simulink model "TAXI"  (R2024b)
settings: Solver=FixedStepDiscrete  StartTime=0.0  StopTime=13  FixedStep=0.01  RelTol=1e-3
settings Model: Creator=A  LastModifiedBy=A
settings OptimizationCC: DefaultParameterBehavior=Inlined  UseDivisionForNetSlopeComputation=on  GainParamInheritBuiltInType=on  UseFloatMulNetSlope=on  InlineInvariantSignals=on  ReuseModelBlockBuffer=off  PassReuseOutputArgsAs=Individual arguments  ZeroExternalMemoryAtStartup=off  ZeroInternalMemoryAtStartup=off  NoFixptDivByZeroProtection=on  EfficientFloat2IntCast=on  LifeSpan=1  OptimizeDataStoreBuffers=off  BusAssignmentInplaceUpdate=off  OptimizationLevel=level0  EfficientTunableParamExpr=on
settings DebuggingCC: ParameterTunabilityLossMsg=error  StrictBusMsg=ErrorOnBusTreatedAsVector  NonBusSignalsTreatedAsBus=error
settings HardwareCC: ProdBitPerPointer=32  ProdBitPerSizeT=32  ProdBitPerPtrDiffT=32  ProdLargestAtomicFloat=None  ProdWordSize=32  ProdLongLongMode=on  ProdHWDeviceType=Infineon->TriCore
settings SFSimCC: MATLABDynamicMemAlloc=off
settings RTWCC: Description=Embedded Coder  SystemTargetFile=ert.tlc  GenCodeOnly=on  TemplateMakefile=ert_default_tmf  GenerateReport=on  LaunchReport=on  DataTypeReplacement=CDataTypesFixedWidth  GenerateCodeMetricsReport=on
settings CodeAppCC: ForceParamTrailComments=on  IgnoreCustomStorageClasses=off  OperatorAnnotations=on  SimulinkDataObjDesc=on  SFDataObjDesc=on  CustomSymbolStrGlobalVar=rt$N$M  CustomSymbolStrType=$N$M  CustomSymbolStrFcn=$N$M$F  CustomSymbolStrMacro=$N$M  InsertBlockDesc=on
settings ERTTargetCC: TargetLangStandard=C99 (ISO)  GenerateSampleERTMain=on  IncludeMdlTerminateFcn=off  CombineSignalStateStructs=on  SupportAbsoluteTime=off  PurelyIntegerCode=on  SupportComplex=off  SupportNonInlinedSFcns=on  ERTCustomFileTemplate=example_file_process.tlc  IndentStyle=Allman  IndentSize=4  MaxIdInt64=INT64_MAX  MinIdInt64=INT64_MIN  MaxIdUint64=UINT64_MAX  MaxIdInt32=INT32_MAX  MinIdInt32=INT32_MIN  MaxIdUint32=UINT32_MAX  MaxIdInt16=INT16_MAX  MinIdInt16=INT16_MIN  MaxIdUint16=UINT16_MAX  MaxIdInt8=INT8_MAX  MinIdInt8=INT8_MIN  MaxIdUint8=UINT8_MAX
settings ConfigComp: CovEnable=on  RecordCoverage=on  CovMetricSettings=dcmwe  CovModelRefEnable=on

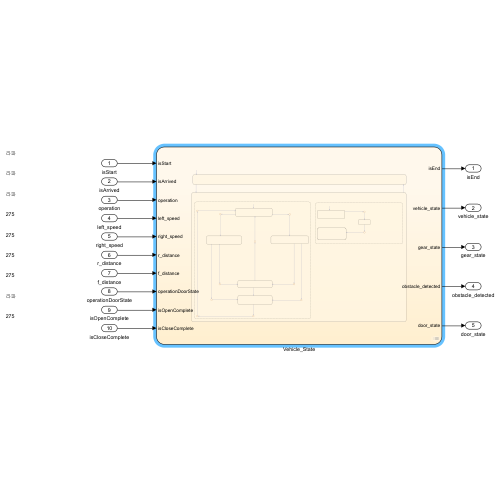
[thumbnail: Simulink's stored preview of the top-level diagram]
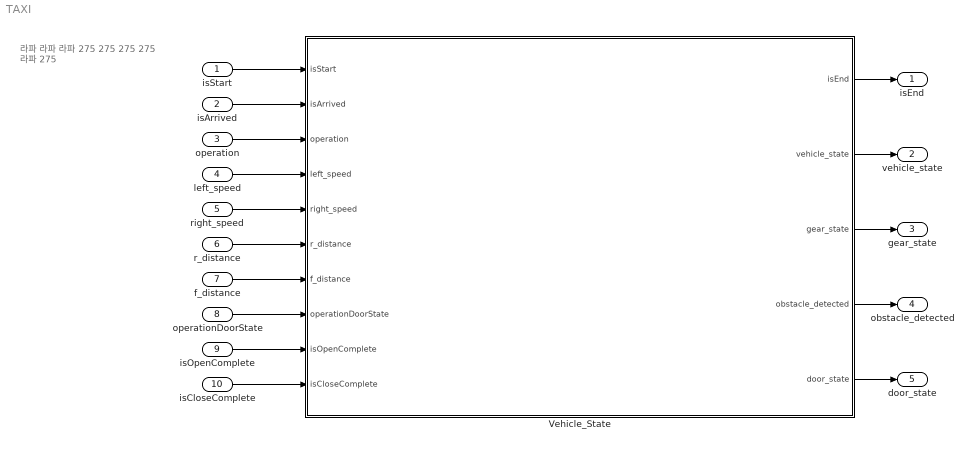
== system TAXI ==
  note: 라파
      |
      |
      | 라파
      |
      |
      | 라파
      |
      |
      | 275
      |
      |
      | 275
      |
      |
      | 275
      |
      |
      | 275
      |
      |
      | 라파
      |
      |
      | 275
  isStart : Inport  Interpolate=off
  isArrived : Inport  Port=2  Interpolate=off
  operation : Inport  Port=3  Interpolate=off
  left_speed : Inport  Port=4  Interpolate=off
  right_speed : Inport  Port=5  Interpolate=off
  r_distance : Inport  Port=6  Interpolate=off
  f_distance : Inport  Port=7  Interpolate=off
  operationDoorState : Inport  Port=8  Interpolate=off
  isOpenComplete : Inport  Port=9  Interpolate=off
  isCloseComplete : Inport  Port=10  Interpolate=off
  Vehicle_State : Stateflow chart  TreatAsAtomicUnit=on  RTWFcnName=State_Control  RTWFileName=Vehicle_State_Controller
      settings: RTWSystemCode=Reusable function  RTWFcnNameOpts=User specified  RTWFileNameOpts=User specified
  isEnd : Outport
  vehicle_state : Outport  Port=2
  gear_state : Outport  Port=3
  obstacle_detected : Outport  Port=4
  door_state : Outport  Port=5
  wires:
  operation/1 -> Vehicle_State/3(operation)
  isArrived/1 -> Vehicle_State/2(isArrived)
  left_speed/1 -> Vehicle_State/4(left_speed)
  right_speed/1 -> Vehicle_State/5(right_speed)
  r_distance/1 -> Vehicle_State/6(r_distance)
  f_distance/1 -> Vehicle_State/7(f_distance)
  operationDoorState/1 -> Vehicle_State/8(operationDoorState)
  isOpenComplete/1 -> Vehicle_State/9(isOpenComplete)
  Vehicle_State/1(isEnd) -> isEnd/1
  Vehicle_State/2(vehicle_state) -> vehicle_state/1
  Vehicle_State/3(gear_state) -> gear_state/1
  Vehicle_State/4(obstacle_detected) -> obstacle_detected/1
  isStart/1 -> Vehicle_State/1(isStart)
  isCloseComplete/1 -> Vehicle_State/10(isCloseComplete)
  Vehicle_State/5(door_state) -> door_state/1

== stateflow chart TAXI/Vehicle_State ==
  state IDLE
    en:
    isEnd=false;
    vehicle_state = Vehicle_State.IDLE;
  state WORK
    en :
    vehicle_state=Vehicle_State.WORK;
    state GEAR [parallel]
      settings: executionOrder=1
      state PARKING
        en :
        obstacle_detected =false;
        gear_state =Gear_State.P;
      state DRIVING
        en :
        gear_state =Gear_State.D;
      state REVERSE
        en :
        gear_state =Gear_State.R;
      state BRAKE
        en :
        gear_state = Gear_State.B;
      state OBSTACLE_DETECTED
        en:
        obstacle_detected =true;
      (default) -> PARKING
      (junction 279) -> PARKING
      (junction 277) -> (junction 279)
      PARKING -> (junction 399) [order 2] : [operation...
          | ==OperationMode.DRIVING]
      PARKING -> (junction 402) [order 1] : [operation...
          | ==OperationMode.REVERSE]
      (junction 399) -> DRIVING
      (junction 402) -> REVERSE
      (junction 238) -> PARKING : [left_speed==0 &&right_speed==0]
      BRAKE -> (junction 238) [order 1] : [operation...
          | ==OperationMode.PARKING]
      REVERSE -> (junction 410) [order 1] : [operation...
          | ==OperationMode.BRKING]
      REVERSE -> (junction 406) [order 2] : [r_distance<=100 ...
          | &&r_distance>10]
      DRIVING -> (junction 404) [order 2] : [f_distance<=100 ...
          | &&f_distance>10]
      DRIVING -> (junction 408) [order 1] : [operation...
          | ==OperationMode.BRKING]
      (junction 408) -> BRAKE
      (junction 410) -> BRAKE
      BRAKE -> OBSTACLE_DETECTED [order 2] : [f_distance < 10 || r_distance < 10]
      (junction 404) -> OBSTACLE_DETECTED
      (junction 406) -> OBSTACLE_DETECTED
      OBSTACLE_DETECTED -> (junction 273) : [f_distance > 100 && r_distance > 100]
      (junction 273) -> (junction 277) : [left_speed==0 && right_speed==0]
    state DOOR [parallel]
      settings: executionOrder=2
      state DOOR_IDLE
        en:door_state=Door_State.CLOSED;
      state DOOR_OPEN
      state DOOR_CLOSE
        if(isCloseComplete==true)
        isEnd = true;
        end
      (default) -> DOOR_IDLE
      DOOR_IDLE -> (junction 160) : [in(GEAR.PARKING) &&isArrived==true]
      (junction 160) -> DOOR_OPEN : [operationDoorState==OperationDoorState.OPEN]
      DOOR_OPEN -> (junction 162) : [isOpenComplete==true...
          | &&in(GEAR.PARKING)]
          | {door_state = Door_State.OPENED;}
      (junction 162) -> DOOR_CLOSE : [operationDoorState==OperationDoorState.CLOSE]
  (default) -> IDLE
  IDLE -> WORK : [isStart==true]
  WORK -> IDLE : [isEnd == true]
  data: isStart input boolean; isArrived input boolean; operation input Enum: OperationMode; left_speed input uint16 [0..5000] =0; right_speed input uint16 [0..5000] =0; r_distance input uint32; f_distance input uint32 [0..300]; operationDoorState input Enum: OperationDoorState; isEnd output boolean =0; vehicle_state output Enum: Vehicle_State =Vehicle_State.IDLE; isOpenComplete input boolean; gear_state output Enum: Gear_State =Gear_State.P; obstacle_detected output boolean =false; isCloseComplete input boolean; door_state output Enum: Door_State
